simulink model "Controller"  (R2023a)
settings: Solver=VariableStepAuto  StartTime=0.0  StopTime=10.0  RelTol=1e-3
settings Model: Creator=ibaad  LastModifiedBy=ibaad

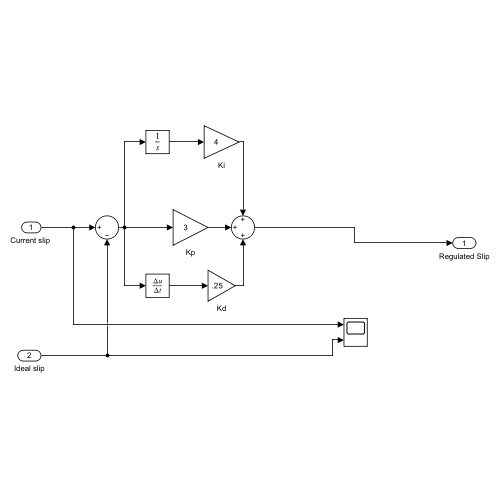
[thumbnail: Simulink's stored preview of the top-level diagram]
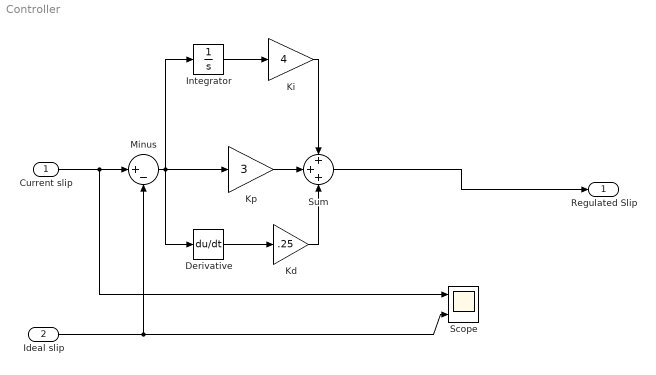
== system Controller ==
  "Current slip " : Inport
  Ideal slip : Inport  Port=2
  Derivative : Derivative
  Integrator : Integrator
  Kd : Gain  Gain=.25
  Ki : Gain  Gain=4
  Kp : Gain  Gain=3
  Minus : Sum  Inputs=|+-
  Scope : Scope  NumInputPorts=2
  Sum : Sum  Inputs=+++
  Regulated Slip : Outport
  wires:
  Kp/1 -> Sum/2
  Sum/1 -> Regulated Slip/1
  Integrator/1 -> Ki/1
  Derivative/1 -> Kd/1
  Ki/1 -> Sum/1
  Kd/1 -> Sum/3
  Ideal slip/1 -> Minus/2, Scope/2
  Minus/1 -> Integrator/1, Kp/1, Derivative/1
  "Current slip "/1 -> Scope/1, Minus/1
